simulink model "Week2_Problem4"  (R2020a)
settings: Solver=VariableStepAuto  StartTime=0.0  StopTime=10  RelTol=1e-3
settings Model: DataDictionary=Week2_Problem4_dic.sldd  Creator=sreeram  LastModifiedBy=sreeram

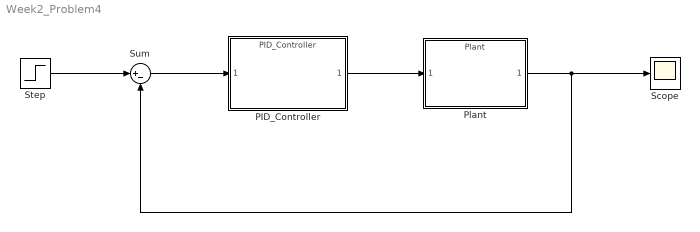
== system Week2_Problem4 ==
  PID_Controller : ModelReference  ModelNameDialog=PID_Controller  ModelReferenceVersion=1.9
  Plant : ModelReference  ModelNameDialog=Plant  ModelReferenceVersion=1.9
  Scope : Scope
  Step : Step  Time=0  Before=1  After=500  SampleTime=0
  Sum : Sum  Inputs=|+-
  wires:
  Step/1 -> Sum/1
  Plant/1 -> Sum/2, Scope/1
  Sum/1 -> PID_Controller/1
  PID_Controller/1 -> Plant/1
